simulink model "Pi"  (R2020b)
settings: Solver=VariableStepAuto  StartTime=0.0  StopTime=10.0  RelTol=1e-3
model workspace (MAT data in the model file):
  K = 0.0247
settings Model: Creator=Diwakar Reddy  LastModifiedBy=Diwakar Reddy
settings DataIOCC: SaveOutput=off  SaveTime=off

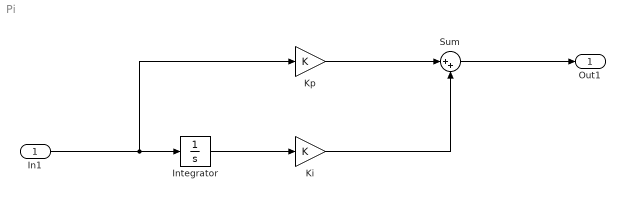
== system Pi ==
  In1 : Inport  OutDataTypeStr=double  PortDimensions=1  SampleTime=0
  Integrator : Integrator
  Ki : Gain  Gain=K
  Kp : Gain  Gain=K
  Sum : Sum  Inputs=|++
  Out1 : Outport  OutDataTypeStr=double  PortDimensions=1  SampleTime=0
  wires:
  Integrator/1 -> Ki/1
  Kp/1 -> Sum/1
  Ki/1 -> Sum/2
  Sum/1 -> Out1/1
  In1/1 -> Integrator/1, Kp/1
